simulink model "FHB_TABS_lib"  (R2013b)
settings: Solver=ode45  StartTime=0.0  StopTime=10.0  RelTol=1e-3
settings Model: Creator=christian.winteler  LastModifiedBy=christian.winteler

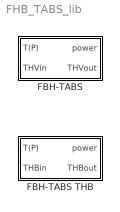
== system FHB_TABS_lib ==
  FBH-TABS : Subsystem  mask(FBH-TABS){d=0.08, d1=0.04, d_pipe=0.015, dr=0.001, dx=0.1, l=70/0.1, lambda_r=0.4, lambda_b=1.4}
      mask prompts: d "thickness of active layer [m]"; d1 "depth of pipes in active layer [m]"; d_pipe "outer diameter of pipes [m]"; dr "wall thickness of pipe [m]"; dx "distance between center of pipes [m]"; l "length of pipe [m]"; lambda_r "conductivity of pipe [W/(m*K)]"; lambda_b "conductivity of layer material [W/(m*K)]"
      mask help:
      | calculates the heating/cooling power from pipes
      | in a floor heating system or a thermally active building component
      | to the active layer in the building element (wall, floor, ceiling)
      | according to the model of M.Koschenz & B.Lehmann, EMPA-CH, 2000
  FBH-TABS THB : Subsystem  mask(FBH-TABS){d=0.08, d1=0.04, d_pipe=0.016, dr=0.002, dx=0.1, l=700, lambda_r=0.35, lambda_b=1.4}
      mask prompts: d "thickness of active layer [m]"; d1 "depth of pipes in active layer [m]"; d_pipe "outer diameter of pipes [m]"; dr "wall thickness of pipe [m]"; dx "distance between center of pipes [m]"; l "length of pipe [m]"; lambda_r "conductivity of pipe [W/(m*K)]"; lambda_b "conductivity of layer material [W/(m*K)]"
      mask help:
      | calculates the heating/cooling power from pipes
      | in a floor heating system or a thermally active building component
      | to the active layer in the building element (wall, floor, ceiling)
      | according to the model of M.Koschenz & B.Lehmann, EMPA-CH, 2000

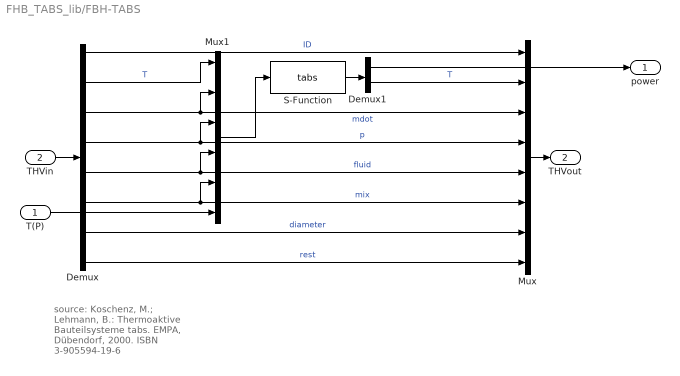
== system FHB_TABS_lib/FBH-TABS ==
  note: source: Koschenz, M.; Lehmann, B.: Thermoaktive Bauteilsysteme tabs. EMPA, Dübendorf, 2000. ISBN 3-905594-19-6
  T(P) : Inport
  THVin : Inport  Port=2
  Demux : Demux  Outputs=[1 1 1 1 1 1 1 13]
  Demux1 : Demux  Outputs=2
  Mux : Mux  Inputs=[1 1 1 1 1 1 1 13]
  Mux1 : Mux  Inputs=6
  S-Function : S-Function  FunctionName=tabs  Parameters=d d1 d_pipe dr dx l lambda_r lambda_b  EnableBusSupport=off
  power : Outport
  THVout : Outport  Port=2  InitialOutput=0
  wires:
  T(P)/1 -> Mux1/6
  Demux1/1 -> power/1
  THVin/1 -> Demux/1
  Demux/2 -> Mux1/1  "T"
  Demux/6 -> Mux1/5, Mux/6  "mix"
  Demux/3 -> Mux1/2, Mux/3  "mdot"
  Demux/7 -> Mux/7  "diameter"
  Demux/8 -> Mux/8  "rest"
  Demux/5 -> Mux1/4, Mux/5  "fluid"
  Demux/1 -> Mux/1  "ID"
  Mux/1 -> THVout/1
  Demux1/2 -> Mux/2  "T"
  Demux/4 -> Mux1/3, Mux/4  "p"
  S-Function/1 -> Demux1/1
  Mux1/1 -> S-Function/1

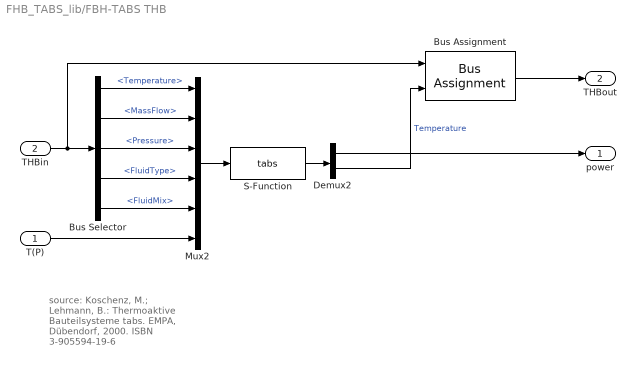
== system FHB_TABS_lib/FBH-TABS THB ==
  note: source: Koschenz, M.; Lehmann, B.: Thermoaktive Bauteilsysteme tabs. EMPA, Dübendorf, 2000. ISBN 3-905594-19-6
  T(P) : Inport
  THBin : Inport  Port=2
  Bus Assignment : BusAssignment  AssignedSignals=Temperature
  Bus Selector : BusSelector  OutputSignals=Temperature,MassFlow,Pressure,FluidType,FluidMix
  Demux2 : Demux  Outputs=2
  Mux2 : Mux  Inputs=6
  S-Function : S-Function  FunctionName=tabs  Parameters=d d1 d_pipe dr dx l lambda_r lambda_b  EnableBusSupport=off
  power : Outport
  THBout : Outport  Port=2  InitialOutput=0
  wires:
  Bus Assignment/1 -> THBout/1
  Demux2/1 -> power/1
  Demux2/2 -> Bus Assignment/2  "Temperature"
  S-Function/1 -> Demux2/1
  Mux2/1 -> S-Function/1
  Bus Selector/1 -> Mux2/1  "<Temperature>"
  Bus Selector/5 -> Mux2/5  "<FluidMix>"
  Bus Selector/2 -> Mux2/2  "<MassFlow>"
  Bus Selector/3 -> Mux2/3  "<Pressure>"
  Bus Selector/4 -> Mux2/4  "<FluidType>"
  THBin/1 -> Bus Selector/1, Bus Assignment/1
  T(P)/1 -> Mux2/6
